simulink model "Fadhlan_Firasyan_Step_Control_Test_2Okt2024"  (R2023a)
settings: Solver=VariableStepAuto  StartTime=0.0  StopTime=10.0  RelTol=1e-3
settings Model: Creator=HP  LastModifiedBy=HP

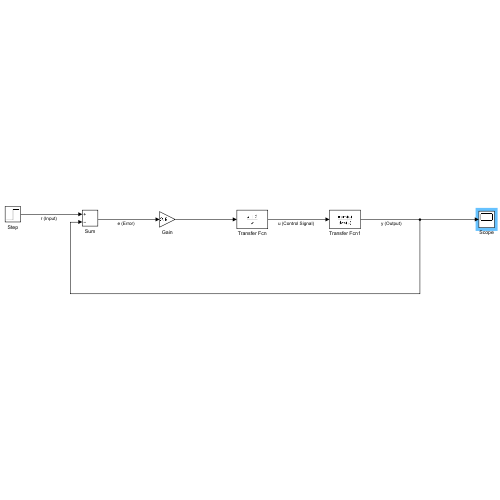
[thumbnail: Simulink's stored preview of the top-level diagram]
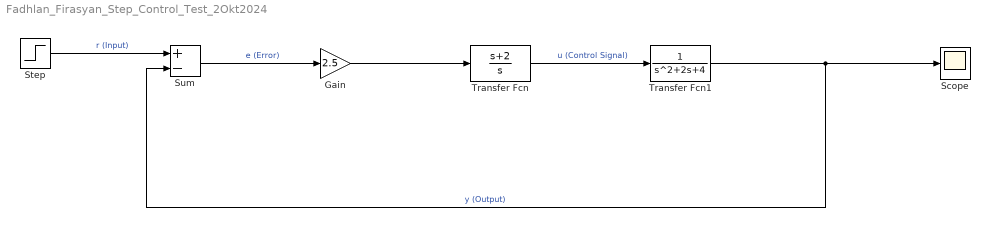
== system Fadhlan_Firasyan_Step_Control_Test_2Okt2024 ==
  Gain : Gain  Gain=2.5
  Scope : Scope
  Step : Step  SampleTime=0
  Sum : Sum  Inputs=+-
  Transfer Fcn : TransferFcn  Numerator=[1 2]  Denominator=[1 0]
  Transfer Fcn1 : TransferFcn  Denominator=[1 2 4]
  wires:
  Step/1 -> Sum/1  "r (Input)"
  Sum/1 -> Gain/1  "e (Error)"
  Gain/1 -> Transfer Fcn/1
  Transfer Fcn/1 -> Transfer Fcn1/1  "u (Control Signal)"
  Transfer Fcn1/1 -> Sum/2, Scope/1  "y (Output)"
